simulink model "ch4f31"  (Simulink 3.00)
settings: Solver=ode45  SolverMode=SingleTasking  StartTime=0.0  StopTime=25  RelTol=1e-3  AbsTol=1e-6
CloseFcn:
  | ;slview('closediagram',bdroot);
settings Model: OptimizeBlockIOStorage=off

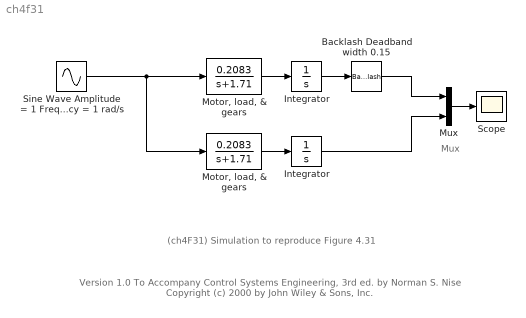
== system ch4f31 ==
  note: Mux
  note: Version 1.0
      | To Accompany Control Systems Engineering, 3rd ed. by Norman S. Nise
      | Copyright (c) 2000 by John Wiley & Sons, Inc.
  note: (ch4F31) Simulation to reproduce Figure 4.31
  Backlash Deadband width 0.15 : Backlash  BacklashWidth=0.15  InitialOutput=0
  Integrator : Integrator  ExternalReset=none  InitialConditionSource=internal  InitialCondition=0  LimitOutput=off  UpperSaturationLimit=inf  LowerSaturationLimit=-inf  ShowSaturationPort=off  ShowStatePort=off  AbsoluteTolerance=auto
  "Integrator " : Integrator  ExternalReset=none  InitialConditionSource=internal  InitialCondition=0  LimitOutput=off  UpperSaturationLimit=inf  LowerSaturationLimit=-inf  ShowSaturationPort=off  ShowStatePort=off  AbsoluteTolerance=auto
  "Motor, load, & gears" : TransferFcn  Numerator=0.2083  Denominator=[1 1.71]
  "Motor, load, & gears " : TransferFcn  Numerator=0.2083  Denominator=[1 1.71]
  Mux : Mux  Inputs=2
  Scope : Scope
      settings: TickLabels=on  TimeRange=25  YMin=0  YMax=0.25  SaveToWorkspace=off  SaveName=ScopeData  DataFormat=Matrix
  Sine Wave Amplitude = 1 Frequency = 1 rad/s : Sin  Amplitude=1  Frequency=1  Phase=0  SampleTime=0
  wires:
  Sine Wave Amplitude = 1 Frequency = 1 rad/s/1 -> "Motor, load, & gears "/1, "Motor, load, & gears"/1
  "Motor, load, & gears"/1 -> Integrator/1
  Integrator/1 -> Backlash Deadband width 0.15/1
  Backlash Deadband width 0.15/1 -> Mux/1
  "Motor, load, & gears "/1 -> "Integrator "/1
  "Integrator "/1 -> Mux/2
  Mux/1 -> Scope/1
